simulink model "walkingRobotInvKin"  (R2020a)
settings: Solver=ode15s  StartTime=0.0  StopTime=10  MaxStep=1e-2  EnableMultiTasking=on
values from neighbouring files (symbols this model uses):
  ankle_servo_kd = 8    [robotParametersInvKin.m]
  ankle_servo_ki = 4    [robotParametersInvKin.m]
  ankle_servo_kp = 20    [robotParametersInvKin.m]
  deriv_filter_coeff = 100    [robotParametersInvKin.m]
  foot_height_offset = sqrt( (lower_leg_length+upper_leg_length)^2                           - ((stepLength/2)*100)^2 ) - 1e-3    [robotParametersInvKin.m]
  foot_x = 8    [robotParametersInvKin.m]
  foot_y = 6    [robotParametersInvKin.m]
  foot_z = 1    [robotParametersInvKin.m]
  gaitPeriod = 0.75    [robotParametersInvKin.m]
  height_plane = 0.025    [robotParametersInvKin.m]
  initAnglesR = init_ang * [1; 0; -1]    [robotParametersInvKin.m]
  joint_stiffness = 1    [robotParametersInvKin.m]
  lower_leg_length = 10    [robotParametersInvKin.m]
  plane_x = 25    [robotParametersInvKin.m]
  plane_y = 3    [robotParametersInvKin.m]
  stepHeight = 0.025    [robotParametersInvKin.m]
  stepLength = 0.075    [robotParametersInvKin.m]
  torso_offset_x = -1    [robotParametersInvKin.m]
  torso_offset_z = -2    [robotParametersInvKin.m]
  torso_x = 5    [robotParametersInvKin.m]
  torso_y = 10    [robotParametersInvKin.m]
  torso_z = 8    [robotParametersInvKin.m]
  upper_leg_length = 10    [robotParametersInvKin.m]
undefined symbols (not defined in the file or in its folder): X, Y, Z
libraries: sm_lib x31, walkingRobotUtils x10, Contact_Forces_Lib x8, nesl_utility x6, simulink x2
(part 2 of 2)

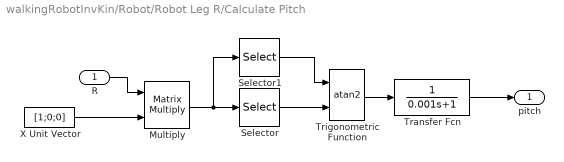
== system walkingRobotInvKin/Robot/Robot Leg R/Calculate Pitch ==
  R : Inport
  Multiply : Product  Multiplication=Matrix(*)
  Selector : Selector  InputPortWidth=3  IndexOptions=Index vector (dialog)  Indices=1  OutputSizes=1
  Selector1 : Selector  InputPortWidth=3  IndexOptions=Index vector (dialog)  Indices=2  OutputSizes=1
  Transfer Fcn : TransferFcn  Denominator=[0.001 1]
  Trigonometric Function : Trigonometry  Operator=atan2
  X Unit Vector : Constant  Value=[1;0;0]
  pitch : Outport
  wires:
  Trigonometric Function/1 -> Transfer Fcn/1
  X Unit Vector/1 -> Multiply/2
  Selector/1 -> Trigonometric Function/2
  R/1 -> Multiply/1
  Selector1/1 -> Trigonometric Function/1
  Multiply/1 -> Selector1/1, Selector/1
  Transfer Fcn/1 -> pitch/1

== matlab function walkingRobotInvKin/Robot/Evaluate Foot Trajectory L ==
  data: t input; x output; y output; stepLength parameter; stepHeight parameter; gaitPeriod parameter
function [x,y] = footTraj(t, stepLength, stepHeight, gaitPeriod)
    
    [x,y] = evalFootGait(t,stepLength,stepHeight,gaitPeriod);

end

== matlab function walkingRobotInvKin/Robot/Leg IK R ==
  data: x input; t1 output; y input; t2 output; foot_height_offset parameter; upper_leg_length parameter; lower_leg_length parameter
function [t1,t2] = invKin2D(x,y, foot_height_offset, upper_leg_length, lower_leg_length)

    % Call symbolic generated function
    theta = legInvKin(upper_leg_length/100,lower_leg_length/100,... 
                      -x,y-foot_height_offset/100);
    
    % Address multiple outputs
    if size(theta,1) == 2
       if theta(1,2) < 0
          t1 = theta(2,1);
          t2 = theta(2,2);
       else
          t1 = theta(1,1);
          t2 = theta(1,2);
       end
    else
        t1 = theta(1);
        t2 = theta(2);
    end
    
end

== matlab function walkingRobotInvKin/Robot/Leg IK L ==
  data: x input; t1 output; y input; t2 output; foot_height_offset parameter; upper_leg_length parameter; lower_leg_length parameter
function [t1,t2] = invKin2D(x,y, foot_height_offset, upper_leg_length, lower_leg_length)

    % Call symbolic generated function
    theta = legInvKin(upper_leg_length/100,lower_leg_length/100,... 
                      -x,y-foot_height_offset/100);
    
    % Address multiple outputs
    if size(theta,1) == 2
       if theta(1,2) < 0
          t1 = theta(2,1);
          t2 = theta(2,2);
       else
          t1 = theta(1,1);
          t2 = theta(1,2);
       end
    else
        t1 = theta(1);
        t2 = theta(2);
    end
    
end

== matlab function walkingRobotInvKin/Robot/Evaluate Foot Trajectory R ==
  settings: sampleTime=0.01
  data: t input; x output; y output; stepLength parameter; stepHeight parameter; gaitPeriod parameter
function [x,y] = footTraj(t, stepLength, stepHeight, gaitPeriod)
    
    [x,y] = evalFootGait(t,stepLength,stepHeight,gaitPeriod);

end
